simulink model "dynamiczny_model_ciagly"  (R2016b)
settings: Solver=ode45  StartTime=0.0  StopTime=100  RelTol=1e-3  EnableMultiTasking=on
values from neighbouring files (symbols this model uses):
  a1 = -0.19    [initial.m]
  a2 = -0.05    [initial.m]
  a3 = -0.95    [initial.m]
  a4 = -0.45    [initial.m]
  K = 5.5    [initial.m]
  T1 = 7    [initial.m]
  T2 = 7    [initial.m]
settings Model: Creator=Agnieszka i Kamilka  LastModifiedBy=kamil
settings DataIOCC: LimitDataPoints=on  SaveFormat=Array  SignalLoggingSaveFormat=ModelDataLogs
settings OptimizationCC: ExpressionDepthLimit=2147483647  LifeSpan=inf
settings DebuggingCC: UnderspecifiedInitializationDetection=Classic  MergeDetectMultiDrivingBlocksExec=none  FcnCallInpInsideContextMsg=warning  StateNameClashWarn=warning  SFUnexpectedBacktrackingDiag=warning  SFNoUnconditionalDefaultTransitionDiag=warning  SFExecutionAtInitializationDiag=none
settings HardwareCC: ProdBitPerPointer=32  ProdBitPerSizeT=32  ProdBitPerPtrDiffT=32  ProdLargestAtomicFloat=None  ProdIntDivRoundTo=Undefined  ProdEndianess=Unspecified  ProdWordSize=32  ProdHWDeviceType=32-bit Generic
settings ModelReferenceCC: PropagateSignalLabelsOutOfModel=off
settings GRTTargetCC: TargetLangStandard=C89/C90 (ANSI)  GeneratePreprocessorConditionals=Disable all  CombineOutputUpdateFcns=off  GRTInterface=on
settings ConfigComp: CovMetricSettings=dw  CovHtmlReporting=on  CovSaveCumulativeToWorkspaceVar=on  CovSaveSingleToWorkspaceVar=on  CovExternalEMLEnable=off

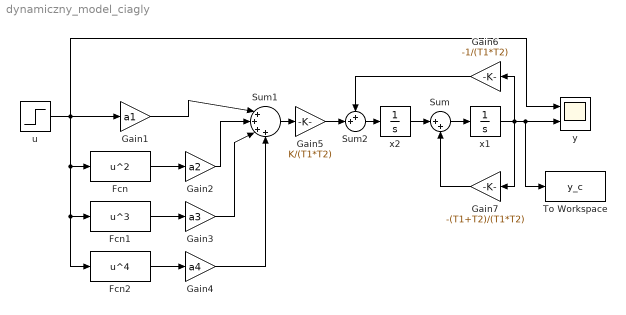
== system dynamiczny_model_ciagly ==
  Fcn : Fcn  Expr=u^2
  Fcn1 : Fcn  Expr=u^3
  Fcn2 : Fcn  Expr=u^4
  "Gain1 " : Gain  Gain=a1
  Gain2 : Gain  Gain=a2
  "Gain3 " : Gain  Gain=a3
  "Gain4 " : Gain  Gain=a4
  Gain5 : Gain  Gain=K/(T1*T2)
  Gain6 : Gain  Gain=-1/(T1*T2)
  Gain7 : Gain  Gain=-(T1+T2)/(T1*T2)
  Sum : Sum  Inputs=|++
  Sum1 : Sum  Inputs=|++++
  Sum2 : Sum  Inputs=++|
  To Workspace : ToWorkspace  VariableName=y_c  SaveFormat=Structure With Time  SampleTime=-1
  "u " : Step  SampleTime=0
  x1 : Integrator
  x2 : Integrator
  y : Scope  NumInputPorts=2
  wires:
  Sum1/1 -> Gain5/1
  "Gain1 "/1 -> Sum1/1
  "u "/1 -> "Gain1 "/1, Fcn2/1, Fcn1/1, Fcn/1, y/1
  Fcn/1 -> Gain2/1
  Fcn1/1 -> "Gain3 "/1
  Fcn2/1 -> "Gain4 "/1
  Gain2/1 -> Sum1/2
  "Gain3 "/1 -> Sum1/3
  "Gain4 "/1 -> Sum1/4
  x2/1 -> Sum/1
  Sum/1 -> x1/1
  x1/1 -> Gain7/1, Gain6/1, y/2, To Workspace/1
  Gain7/1 -> Sum/2
  Gain6/1 -> Sum2/1
  Gain5/1 -> Sum2/2
  Sum2/1 -> x2/1
